simulink model "EngDem_TrqLimCoord"  (R2016b)
settings: configuration reference "CodeGenConfigSet" (kept outside this file)
values from neighbouring files (symbols this model uses):
  EngDem_facAdj_C = Calibration.Parameter    [init_EngDem_TrqLimCoord.m]    (also in init_EngDem_TrqLimCoord_SIL.m = Simulink.Parameter)
  EngDem_facAdjMax_C = Calibration.Parameter    [init_EngDem_TrqLimCoord.m]    (also in init_EngDem_TrqLimCoord_SIL.m = Simulink.Parameter)
  EngDem_facAdjMin_C = Calibration.Parameter    [init_EngDem_TrqLimCoord.m]    (also in init_EngDem_TrqLimCoord_SIL.m = Simulink.Parameter)
  EngDem_facDvolPT1_C = Calibration.Parameter    [init_EngDem_TrqLimCoord.m]    (also in init_EngDem_TrqLimCoord_SIL.m = Simulink.Parameter)
  EngDem_facResFlowPT1_C = Calibration.Parameter    [init_EngDem_TrqLimCoord.m]    (also in init_EngDem_TrqLimCoord_SIL.m = Simulink.Parameter)
  EngDem_RmpLimErrNeg_C = Calibration.Parameter    [init_EngDem_TrqLimCoord.m]    (also in init_EngDem_TrqLimCoord_SIL.m = Simulink.Parameter)
  EngDem_RmpLimErrPos_C = Calibration.Parameter    [init_EngDem_TrqLimCoord.m]    (also in init_EngDem_TrqLimCoord_SIL.m = Simulink.Parameter)
  EngDem_trqLimErr1_CUR = Calibration.Parameter    [init_EngDem_TrqLimCoord.m]    (also in init_EngDem_TrqLimCoord_SIL.m = Simulink.Parameter)
  EngDem_trqLimErr1_CURX = Calibration.Parameter    [init_EngDem_TrqLimCoord.m]    (also in init_EngDem_TrqLimCoord_SIL.m = Simulink.Parameter)
  EngDem_trqLimErr2_CUR = Calibration.Parameter    [init_EngDem_TrqLimCoord.m]    (also in init_EngDem_TrqLimCoord_SIL.m = Simulink.Parameter)
  EngDem_trqLimErr2_CURX = Calibration.Parameter    [init_EngDem_TrqLimCoord.m]    (also in init_EngDem_TrqLimCoord_SIL.m = Simulink.Parameter)
  EngDem_trqLimErr3_CUR = Calibration.Parameter    [init_EngDem_TrqLimCoord.m]    (also in init_EngDem_TrqLimCoord_SIL.m = Simulink.Parameter)
  EngDem_trqLimErr3_CURX = Calibration.Parameter    [init_EngDem_TrqLimCoord.m]    (also in init_EngDem_TrqLimCoord_SIL.m = Simulink.Parameter)
  EngDem_trqLimErr4_CUR = Calibration.Parameter    [init_EngDem_TrqLimCoord.m]    (also in init_EngDem_TrqLimCoord_SIL.m = Simulink.Parameter)
  EngDem_trqLimErr4_CURX = Calibration.Parameter    [init_EngDem_TrqLimCoord.m]    (also in init_EngDem_TrqLimCoord_SIL.m = Simulink.Parameter)
  EngDem_TrqLimErrRmpNeg_C = Calibration.Parameter    [init_EngDem_TrqLimCoord.m]    (also in init_EngDem_TrqLimCoord_SIL.m = Simulink.Parameter)
  EngDem_TrqLimErrRmpPos_C = Calibration.Parameter    [init_EngDem_TrqLimCoord.m]    (also in init_EngDem_TrqLimCoord_SIL.m = Simulink.Parameter)
  EngDem_trqLimPDiff_CUR = Calibration.Parameter    [init_EngDem_TrqLimCoord.m]    (also in init_EngDem_TrqLimCoord_SIL.m = Simulink.Parameter)
  EngDem_trqLimPDiff_CURX = Calibration.Parameter    [init_EngDem_TrqLimCoord.m]    (also in init_EngDem_TrqLimCoord_SIL.m = Simulink.Parameter)
  TRQ_MAX = fi(1000,Trq_Nm)    [init_EngDem_TrqLimCoord.m]    (also in init_EngDem_TrqLimCoord_SIL.m)
undefined symbols (not defined in the file or in its folder): CEngDsT_tTransf_CURX, EngDem_TrqLimCoord_DT
libraries: CXLib x9, simulink x1
settings Model: Creator=Administrator  LastModifiedBy=bianxuyin
settings ConfigSetRef: SourceLocation=Base Workspace

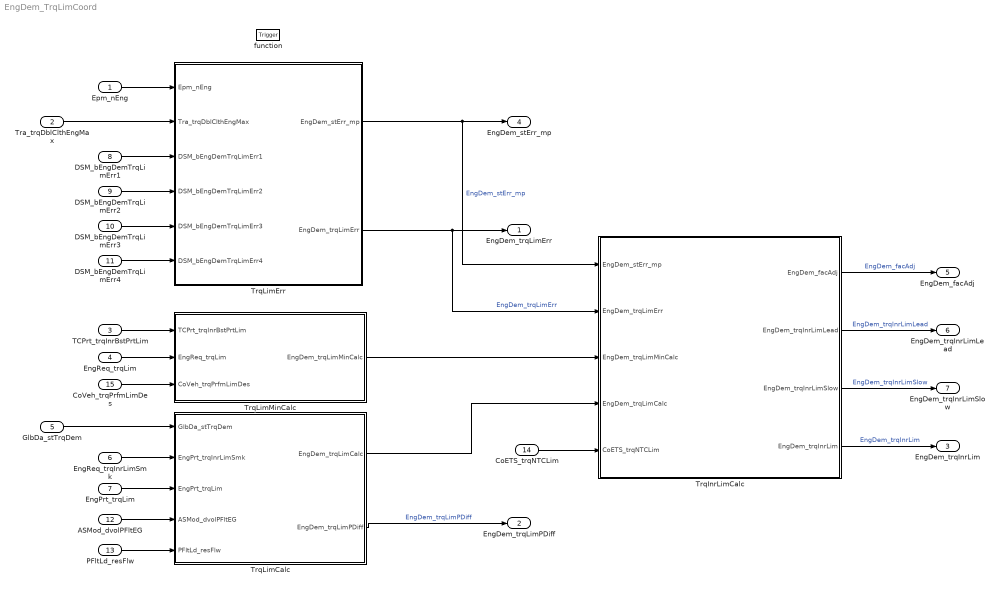
== system EngDem_TrqLimCoord ==
  Epm_nEng : Inport  Tag=rpm  Description=Engine speed  OutMin=0  OutMax=6000  OutDataTypeStr=EngSpeed_rpm
  Tra_trqDblClthEngMax : Inport  Tag=Nm  Description=Application parameter for minimum torque of systemdegratation Nm  Port=2  OutMin=-3000  OutMax=3000  OutDataTypeStr=Trq_Nm
  TCPrt_trqInrBstPrtLim : Inport  Tag=Nm  Description=Torque limitation from VGT Nm  Port=3  OutMin=-3276.8  OutMax=3276.7  OutDataTypeStr=Trq_Nm
  EngReq_trqLim : Inport  Tag=Nm  Description=Resulting limiting torque from engine specifications  Port=4  OutMin=-3276.8  OutMax=3276.7  OutDataTypeStr=Trq_Nm
  GlbDa_stTrqDem : Inport  Description=contains highest prior function with torque demand  Port=5  OutMin=0  OutMax=4294967295  OutDataTypeStr=State_uint32
  EngReq_trqInrLimSmk : Inport  Tag=Nm  Description=Limiting torque smoke limit  Port=6  OutMin=-3276.8  OutMax=3276.7  OutDataTypeStr=Trq_Nm
  EngPrt_trqLim : Inport  Tag=Nm  Description=Limitation torque for engine mechanic protection by torque limitation (as inner engine torque)  Port=7  OutMin=-3276.8  OutMax=3276.7  OutDataTypeStr=Trq_Nm
  DSM_bEngDemTrqLimErr1 : Inport  Description=FId for Engine demand Torque Limitation due to System error  Port=8  OutMin=0  OutMax=1  OutDataTypeStr=boolean
  DSM_bEngDemTrqLimErr2 : Inport  Description=FId for Engine demand Torque Limitation due to System error  Port=9  OutMin=0  OutMax=1  OutDataTypeStr=boolean
  DSM_bEngDemTrqLimErr3 : Inport  Description=FId for Engine demand Torque Limitation due to System error  Port=10  OutMin=0  OutMax=1  OutDataTypeStr=boolean
  DSM_bEngDemTrqLimErr4 : Inport  Description=FId for Engine demand Torque Limitation due to System error  Port=11  OutMin=0  OutMax=1  OutDataTypeStr=boolean
  ASMod_dvolPFltEG : Inport  Tag=m^3/h  Description=Calculated exhaust-gas volume flow in the particulate filter  Port=12  OutMin=0  OutMax=100  OutDataTypeStr=AirVol_m3_h
  PFltLd_resFlw : Inport  Tag=kPa/(m^3/h)  Description=Flow resistance of the particulate filter  Port=13  OutMin=-0.3  OutMax=0.3  OutDataTypeStr=FlowRes_kPa_m3_h
  CoETS_trqNTCLim : Inport  Tag=Nm  Description=NTC torque limitation (0 in braking, ramped to max in braked to fired  Port=14  OutMin=0  OutMax=1000  OutDataTypeStr=Trq_Nm
  CoVeh_trqPrfmLimDes : Inport  Tag=Nm  Description=Torque limitation from performence limiter  Port=15  OutMin=-3000  OutMax=3276.7  OutDataTypeStr=Trq_Nm
  function : TriggerPort  TriggerType=function-call  VariantControl=Variant
  TrqInrLimCalc : Subsystem
  TrqLimCalc : Subsystem  RTWFcnName=TrqLimCalc_Co  RTWFileName=TrqLimCalc
      settings: RTWSystemCode=Nonreusable function  RTWFcnNameOpts=User specified  RTWFileNameOpts=User specified
  TrqLimErr : Subsystem  RTWFcnName=TrqLimErr_Co  RTWFileName=TrqLimErr
      settings: RTWSystemCode=Nonreusable function  RTWFcnNameOpts=User specified  RTWFileNameOpts=User specified
  TrqLimMinCalc : Subsystem  RTWFcnName=TrqLimMinCalc_Co  RTWFileName=TrqLimMinCalc
      settings: RTWSystemCode=Nonreusable function  RTWFcnNameOpts=User specified  RTWFileNameOpts=User specified
  EngDem_trqLimErr : Outport  Tag=Nm  Description=Substitute limiting torque in the event of an error  OutMin=-3276.8  OutMax=3276.7  OutDataTypeStr=Trq_Nm
  EngDem_trqLimPDiff : Outport  Tag=Nm  Description=Limiting torque due to exhaust gas back-pressure  Port=2  OutMin=-3276.8  OutMax=3276.7  OutDataTypeStr=Trq_Nm
  EngDem_trqInrLim : Outport  Tag=Nm  Description=Resulting limiting torque (inner engine torque)  Port=3  OutMin=-3276.8  OutMax=3276.7  OutDataTypeStr=Trq_Nm
  EngDem_stErr_mp : Outport  Description=Status of the limitation FIDs  Port=4  OutMin=0  OutMax=1  OutDataTypeStr=boolean
  EngDem_facAdj : Outport  Description=EEPROM adjustment value for correction of the limiting torque  Port=5  OutMin=-10  OutMax=10  OutDataTypeStr=Factor
  EngDem_trqInrLimLead : Outport  Tag=Nm  Description=inner engine limted lead torque  Port=6  OutMin=-3276.8  OutMax=3276.7  OutDataTypeStr=Trq_Nm
  EngDem_trqInrLimSlow : Outport  Tag=Nm  Description=inner engine limted torque for Slow Path  Port=7  OutMin=-3276.8  OutMax=3276.7  OutDataTypeStr=Trq_Nm
  wires:
  TrqLimCalc/2(EngDem_trqLimPDiff) -> EngDem_trqLimPDiff/1  "EngDem_trqLimPDiff"
  Epm_nEng/1 -> TrqLimErr/1(Epm_nEng)
  Tra_trqDblClthEngMax/1 -> TrqLimErr/2(Tra_trqDblClthEngMax)
  TCPrt_trqInrBstPrtLim/1 -> TrqLimMinCalc/1(TCPrt_trqInrBstPrtLim)
  EngReq_trqLim/1 -> TrqLimMinCalc/2(EngReq_trqLim)
  GlbDa_stTrqDem/1 -> TrqLimCalc/1(GlbDa_stTrqDem)
  EngReq_trqInrLimSmk/1 -> TrqLimCalc/2(EngPrt_trqInrLimSmk)
  EngPrt_trqLim/1 -> TrqLimCalc/3(EngPrt_trqLim)
  DSM_bEngDemTrqLimErr1/1 -> TrqLimErr/3(DSM_bEngDemTrqLimErr1)
  DSM_bEngDemTrqLimErr2/1 -> TrqLimErr/4(DSM_bEngDemTrqLimErr2)
  DSM_bEngDemTrqLimErr3/1 -> TrqLimErr/5(DSM_bEngDemTrqLimErr3)
  DSM_bEngDemTrqLimErr4/1 -> TrqLimErr/6(DSM_bEngDemTrqLimErr4)
  TrqLimErr/2(EngDem_trqLimErr) -> EngDem_trqLimErr/1, TrqInrLimCalc/2(EngDem_trqLimErr)  "EngDem_trqLimErr"
  TrqLimMinCalc/1(EngDem_trqLimMinCalc) -> TrqInrLimCalc/3(EngDem_trqLimMinCalc)
  TrqLimCalc/1(EngDem_trqLimCalc) -> TrqInrLimCalc/4(EngDem_trqLimCalc)
  TrqLimErr/1(EngDem_stErr_mp) -> EngDem_stErr_mp/1, TrqInrLimCalc/1(EngDem_stErr_mp)  "EngDem_stErr_mp"
  TrqInrLimCalc/1(EngDem_facAdj) -> EngDem_facAdj/1  "EngDem_facAdj"
  TrqInrLimCalc/4(EngDem_trqInrLim) -> EngDem_trqInrLim/1  "EngDem_trqInrLim"
  TrqInrLimCalc/3(EngDem_trqInrLimSlow) -> EngDem_trqInrLimSlow/1  "EngDem_trqInrLimSlow"
  TrqInrLimCalc/2(EngDem_trqInrLimLead) -> EngDem_trqInrLimLead/1  "EngDem_trqInrLimLead"
  CoVeh_trqPrfmLimDes/1 -> TrqLimMinCalc/3(CoVeh_trqPrfmLimDes)
  ASMod_dvolPFltEG/1 -> TrqLimCalc/4(ASMod_dvolPFltEG)
  PFltLd_resFlw/1 -> TrqLimCalc/5(PFltLd_resFlw)
  CoETS_trqNTCLim/1 -> TrqInrLimCalc/5(CoETS_trqNTCLim)

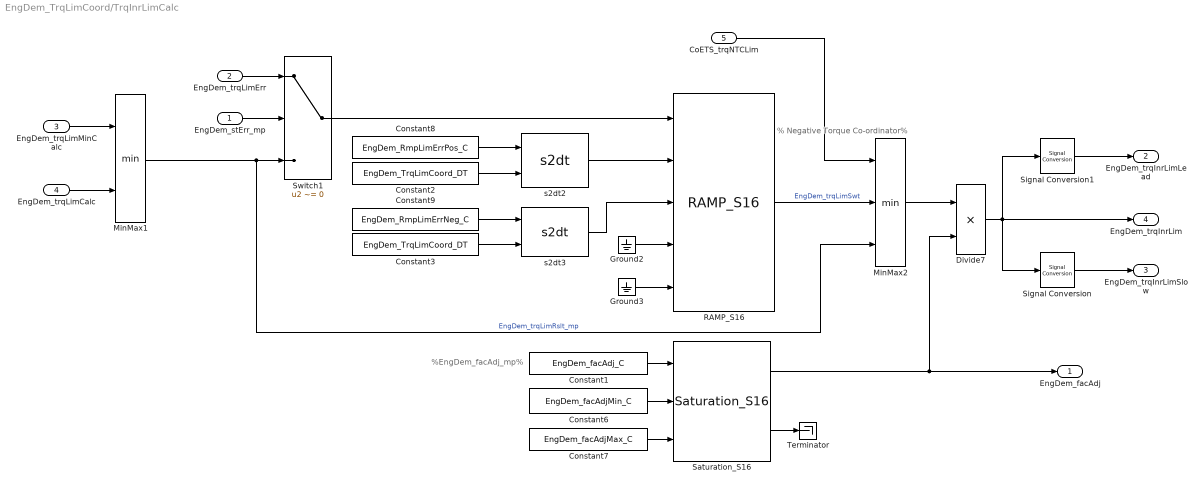
== system EngDem_TrqLimCoord/TrqInrLimCalc ==
  note: % Negative Torque Co-ordinator%
  note: %EngDem_facAdj_mp%
  EngDem_stErr_mp : Inport
  EngDem_trqLimErr : Inport  Port=2
  EngDem_trqLimMinCalc : Inport  Port=3
  EngDem_trqLimCalc : Inport  Port=4
  CoETS_trqNTCLim : Inport  Tag=Nm  Description=NTC torque limitation (0 in braking, ramped to max in braked to fired  Port=5
  Constant1 : Constant  Value=EngDem_facAdj_C
  Constant2 : Constant  Value=EngDem_TrqLimCoord_DT  OutDataTypeStr=Inherit: Inherit via back propagation
  Constant3 : Constant  Value=EngDem_TrqLimCoord_DT  OutDataTypeStr=Inherit: Inherit via back propagation
  Constant6 : Constant  Value=EngDem_facAdjMin_C
  Constant7 : Constant  Value=EngDem_facAdjMax_C
  Constant8 : Constant  Value=EngDem_RmpLimErrPos_C
  Constant9 : Constant  Value=EngDem_RmpLimErrNeg_C
  Divide7 : Product  Inputs=**  OutDataTypeStr=Trq_Nm
  Ground2 : Ground
  Ground3 : Ground
  MinMax1 : MinMax  Inputs=2  InputSameDT=on
  MinMax2 : MinMax  Inputs=3  InputSameDT=on
  RAMP_S16 : CXLib/RAMP_S16
  Saturation_S16 : CXLib/Saturation_S16
  Signal Conversion : SignalConversion  OverrideOpt=off
  Signal Conversion1 : SignalConversion  OverrideOpt=off
  Switch1 : Switch  Criteria=u2 ~= 0  InputSameDT=on
  Terminator : Terminator
  s2dt2 : CXLib/s2dt
  s2dt3 : CXLib/s2dt
  EngDem_facAdj : Outport
  EngDem_trqInrLimLead : Outport  Port=2
  EngDem_trqInrLimSlow : Outport  Port=3
  EngDem_trqInrLim : Outport  Port=4
  wires:
  Ground2/1 -> RAMP_S16/4
  MinMax2/1 -> Divide7/1
  MinMax1/1 -> MinMax2/3, Switch1/3  "EngDem_trqLimRslt_mp"
  EngDem_trqLimCalc/1 -> MinMax1/2
  Constant1/1 -> Saturation_S16/1
  Ground3/1 -> RAMP_S16/5
  Constant6/1 -> Saturation_S16/2
  CoETS_trqNTCLim/1 -> MinMax2/1
  EngDem_trqLimMinCalc/1 -> MinMax1/1
  Saturation_S16/2 -> Terminator/1
  Constant7/1 -> Saturation_S16/3
  Saturation_S16/1 -> EngDem_facAdj/1, Divide7/2
  RAMP_S16/1 -> MinMax2/2  "EngDem_trqLimSwt"
  Constant9/1 -> s2dt3/1
  Constant8/1 -> s2dt2/1
  Switch1/1 -> RAMP_S16/1
  EngDem_trqLimErr/1 -> Switch1/1
  EngDem_stErr_mp/1 -> Switch1/2
  s2dt2/1 -> RAMP_S16/2
  Constant2/1 -> s2dt2/2
  s2dt3/1 -> RAMP_S16/3
  Constant3/1 -> s2dt3/2
  Divide7/1 -> EngDem_trqInrLim/1, Signal Conversion/1, Signal Conversion1/1
  Signal Conversion1/1 -> EngDem_trqInrLimLead/1
  Signal Conversion/1 -> EngDem_trqInrLimSlow/1

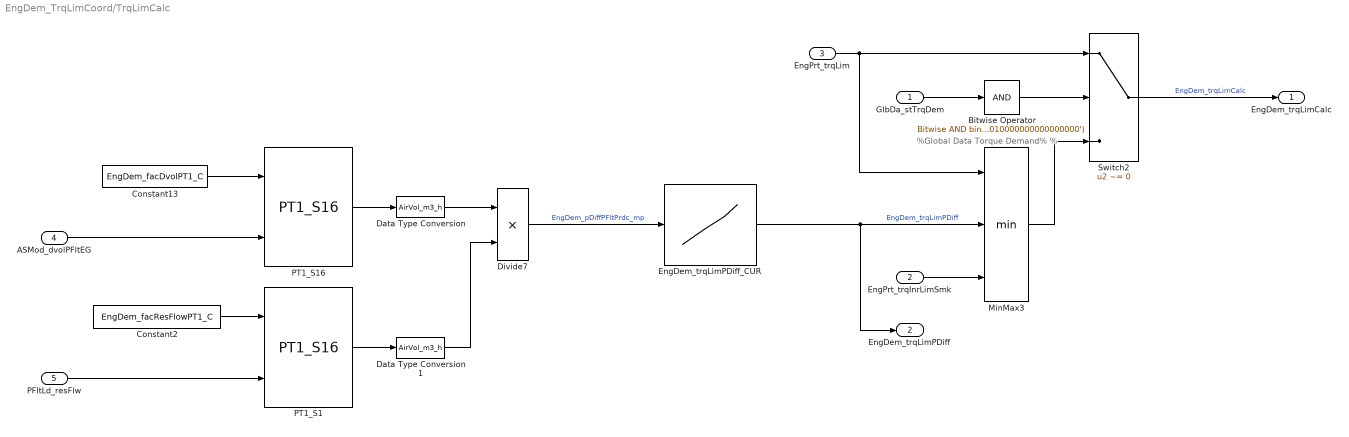
== system EngDem_TrqLimCoord/TrqLimCalc ==
  note: %Global Data Torque Demand% %
  GlbDa_stTrqDem : Inport
  EngPrt_trqInrLimSmk : Inport  Port=2
  EngPrt_trqLim : Inport  Port=3
  ASMod_dvolPFltEG : Inport  Tag=m^2/h  Description=Calculated exhaust-gas volume flow in the particulate filter  Port=4
  PFltLd_resFlw : Inport  Tag=kPa/(m^2/h)  Description=Flow resistance of the particulate filter  Port=5
  " EngDem_trqLimPDiff_CUR" : Lookup_n-D  DialogController=Simulink.DDGSource  NumberOfTableDimensions=1  BreakpointsForDimension1=EngDem_trqLimPDiff_CURX  BreakpointsForDimension2=CEngDsT_tTransf_CURX  IndexSearchMethod=Linear search  BeginIndexSearchUsingPreviousIndexResult=on  Table=EngDem_trqLimPDiff_CUR  ExtrapMethod=Clip  UseLastTableValue=on  InternalRulePriority=Speed  OutDataTypeStr=Inherit: Inherit via back propagation  SaturateOnIntegerOverflow=on
  Bitwise Operator : simulink/Logic and Bit Operations/Bitwise Operator  logicop=AND  UseBitMask=on  BitMask=bin2dec('00000000000000010000000000000000')  BitMaskRealWorld=Stored Integer
  Constant13 : Constant  Value=EngDem_facDvolPT1_C
  Constant2 : Constant  Value=EngDem_facResFlowPT1_C
  Data Type Conversion : DataTypeConversion  OutDataTypeStr=AirVol_m3_h  RndMeth=Round  SaturateOnIntegerOverflow=on
  Data Type Conversion1 : DataTypeConversion  OutDataTypeStr=AirVol_m3_h  RndMeth=Round  SaturateOnIntegerOverflow=on
  Divide7 : Product  Inputs=**  OutDataTypeStr=AirPressure_kPa
  MinMax3 : MinMax  Inputs=3  InputSameDT=on
  PT1_S1 : CXLib/PT1_S16
  PT1_S16 : CXLib/PT1_S16
  Switch2 : Switch  Criteria=u2 ~= 0  InputSameDT=on
  EngDem_trqLimCalc : Outport
  EngDem_trqLimPDiff : Outport  Port=2
  wires:
  GlbDa_stTrqDem/1 -> Bitwise Operator/1
  EngPrt_trqLim/1 -> MinMax3/1, Switch2/1
  MinMax3/1 -> Switch2/3
  " EngDem_trqLimPDiff_CUR"/1 -> EngDem_trqLimPDiff/1, MinMax3/2  "EngDem_trqLimPDiff"
  Divide7/1 -> " EngDem_trqLimPDiff_CUR"/1  "EngDem_pDiffPFltPrdc_mp"
  ASMod_dvolPFltEG/1 -> PT1_S16/2
  EngPrt_trqInrLimSmk/1 -> MinMax3/3
  Switch2/1 -> EngDem_trqLimCalc/1  "EngDem_trqLimCalc"
  Constant13/1 -> PT1_S16/1
  Constant2/1 -> PT1_S1/1
  Bitwise Operator/1 -> Switch2/2
  PT1_S16/1 -> Data Type Conversion/1
  PFltLd_resFlw/1 -> PT1_S1/2
  PT1_S1/1 -> Data Type Conversion1/1
  Data Type Conversion1/1 -> Divide7/2
  Data Type Conversion/1 -> Divide7/1

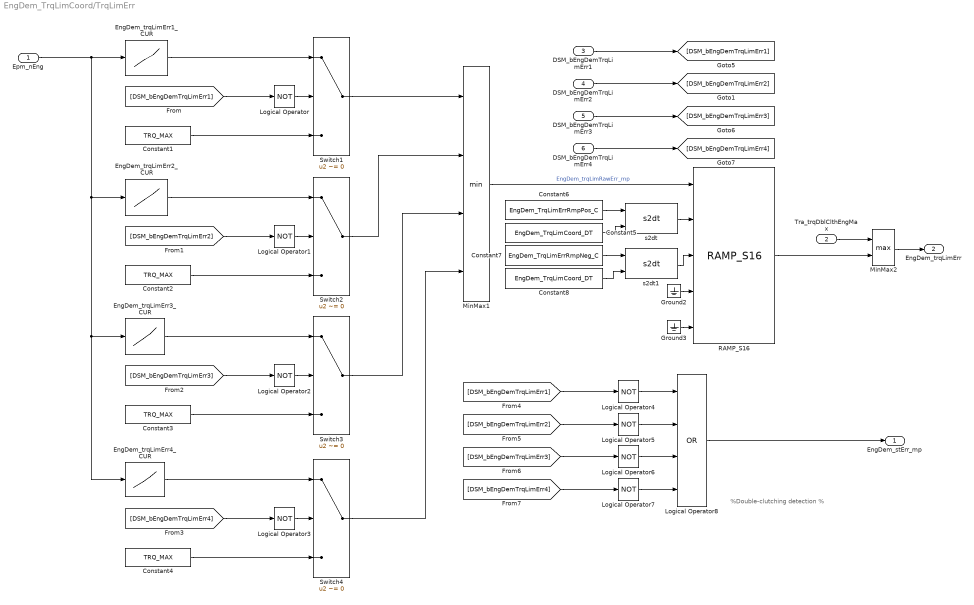
== system EngDem_TrqLimCoord/TrqLimErr ==
  note: %Double-clutching detection %
  Epm_nEng : Inport  Description=Engine speed
  Tra_trqDblClthEngMax : Inport  Port=2
  DSM_bEngDemTrqLimErr1 : Inport  Description=status of FId_EngDemTrqLimErr1  Port=3  OutMin=0  OutMax=1  OutDataTypeStr=boolean
  DSM_bEngDemTrqLimErr2 : Inport  Description=status of FId_EngDemTrqLimErr2  Port=4  OutMin=0  OutMax=1  OutDataTypeStr=boolean
  DSM_bEngDemTrqLimErr3 : Inport  Description=status of FId_EngDemTrqLimErr3  Port=5  OutMin=0  OutMax=1  OutDataTypeStr=boolean
  DSM_bEngDemTrqLimErr4 : Inport  Description=status of FId_EngDemTrqLimErr4  Port=6  OutMin=0  OutMax=1  OutDataTypeStr=boolean
  " EngDem_trqLimErr1_CUR" : Lookup_n-D  DialogController=Simulink.DDGSource  NumberOfTableDimensions=1  BreakpointsForDimension1=EngDem_trqLimErr1_CURX  BreakpointsForDimension2=CEngDsT_tTransf_CURX  IndexSearchMethod=Linear search  BeginIndexSearchUsingPreviousIndexResult=on  Table=EngDem_trqLimErr1_CUR  ExtrapMethod=Clip  UseLastTableValue=on  InternalRulePriority=Speed  OutDataTypeStr=Inherit: Inherit via back propagation  SaturateOnIntegerOverflow=on
  " EngDem_trqLimErr2_CUR" : Lookup_n-D  DialogController=Simulink.DDGSource  NumberOfTableDimensions=1  BreakpointsForDimension1=EngDem_trqLimErr2_CURX  BreakpointsForDimension2=CEngDsT_tTransf_CURX  IndexSearchMethod=Linear search  BeginIndexSearchUsingPreviousIndexResult=on  Table=EngDem_trqLimErr2_CUR  ExtrapMethod=Clip  UseLastTableValue=on  InternalRulePriority=Speed  OutDataTypeStr=Inherit: Inherit via back propagation  SaturateOnIntegerOverflow=on
  " EngDem_trqLimErr3_CUR" : Lookup_n-D  DialogController=Simulink.DDGSource  NumberOfTableDimensions=1  BreakpointsForDimension1=EngDem_trqLimErr3_CURX  BreakpointsForDimension2=CEngDsT_tTransf_CURX  IndexSearchMethod=Linear search  BeginIndexSearchUsingPreviousIndexResult=on  Table=EngDem_trqLimErr3_CUR  ExtrapMethod=Clip  UseLastTableValue=on  InternalRulePriority=Speed  OutDataTypeStr=Inherit: Inherit via back propagation  SaturateOnIntegerOverflow=on
  " EngDem_trqLimErr4_CUR" : Lookup_n-D  DialogController=Simulink.DDGSource  NumberOfTableDimensions=1  BreakpointsForDimension1=EngDem_trqLimErr4_CURX  BreakpointsForDimension2=CEngDsT_tTransf_CURX  IndexSearchMethod=Linear search  BeginIndexSearchUsingPreviousIndexResult=on  Table=EngDem_trqLimErr4_CUR  ExtrapMethod=Clip  UseLastTableValue=on  InternalRulePriority=Speed  OutDataTypeStr=Inherit: Inherit via back propagation  SaturateOnIntegerOverflow=on
  Constant{1..4} (4 alike) : Constant  Value=TRQ_MAX  OutDataTypeStr=Trq_Nm
  Constant5 : Constant  Value=EngDem_TrqLimCoord_DT  OutDataTypeStr=Inherit: Inherit via back propagation
  Constant6 : Constant  Value=EngDem_TrqLimErrRmpPos_C
  Constant7 : Constant  Value=EngDem_TrqLimErrRmpNeg_C
  Constant8 : Constant  Value=EngDem_TrqLimCoord_DT  OutDataTypeStr=Inherit: Inherit via back propagation
  Ground2 : Ground
  Ground3 : Ground
  Logical Operator{,1..7} (8 alike) : Logic  Operator=NOT  AllPortsSameDT=off  OutDataTypeStr=boolean
  Logical Operator8 : Logic  Operator=OR  Inputs=4  AllPortsSameDT=off  OutDataTypeStr=boolean
  MinMax1 : MinMax  Inputs=4  InputSameDT=on
  MinMax2 : MinMax  Function=max  Inputs=2  InputSameDT=on
  RAMP_S16 : CXLib/RAMP_S16
  Switch{1..4} (4 alike) : Switch  Criteria=u2 ~= 0  InputSameDT=on
  s2dt : CXLib/s2dt
  s2dt1 : CXLib/s2dt
  EngDem_stErr_mp : Outport
  EngDem_trqLimErr : Outport  Port=2
  wires:
  MinMax1/1 -> RAMP_S16/1  "EngDem_trqLimRawErr_mp"
  Switch1/1 -> MinMax1/1
  Logical Operator/1 -> Switch1/2
  [DSM_bEngDemTrqLimErr1] -> Logical Operator/1
  " EngDem_trqLimErr1_CUR"/1 -> Switch1/1
  Logical Operator1/1 -> Switch2/2
  [DSM_bEngDemTrqLimErr2] -> Logical Operator1/1
  " EngDem_trqLimErr2_CUR"/1 -> Switch2/1
  Switch2/1 -> MinMax1/2
  Logical Operator2/1 -> Switch3/2
  [DSM_bEngDemTrqLimErr3] -> Logical Operator2/1
  " EngDem_trqLimErr3_CUR"/1 -> Switch3/1
  Switch3/1 -> MinMax1/3
  Logical Operator3/1 -> Switch4/2
  [DSM_bEngDemTrqLimErr4] -> Logical Operator3/1
  " EngDem_trqLimErr4_CUR"/1 -> Switch4/1
  Switch4/1 -> MinMax1/4
  Epm_nEng/1 -> " EngDem_trqLimErr4_CUR"/1, " EngDem_trqLimErr3_CUR"/1, " EngDem_trqLimErr2_CUR"/1, " EngDem_trqLimErr1_CUR"/1
  Ground2/1 -> RAMP_S16/4
  Ground3/1 -> RAMP_S16/5
  Tra_trqDblClthEngMax/1 -> MinMax2/1
  Logical Operator4/1 -> Logical Operator8/1
  Logical Operator5/1 -> Logical Operator8/2
  Logical Operator6/1 -> Logical Operator8/3
  Logical Operator7/1 -> Logical Operator8/4
  Constant6/1 -> s2dt/1
  Constant7/1 -> s2dt1/1
  RAMP_S16/1 -> MinMax2/2
  Logical Operator8/1 -> EngDem_stErr_mp/1
  Constant1/1 -> Switch1/3
  Constant2/1 -> Switch2/3
  Constant3/1 -> Switch3/3
  Constant4/1 -> Switch4/3
  DSM_bEngDemTrqLimErr1/1 -> [DSM_bEngDemTrqLimErr1]
  DSM_bEngDemTrqLimErr2/1 -> [DSM_bEngDemTrqLimErr2]
  DSM_bEngDemTrqLimErr3/1 -> [DSM_bEngDemTrqLimErr3]
  DSM_bEngDemTrqLimErr4/1 -> [DSM_bEngDemTrqLimErr4]
  [DSM_bEngDemTrqLimErr1] -> Logical Operator4/1
  [DSM_bEngDemTrqLimErr2] -> Logical Operator5/1
  [DSM_bEngDemTrqLimErr3] -> Logical Operator6/1
  [DSM_bEngDemTrqLimErr4] -> Logical Operator7/1
  MinMax2/1 -> EngDem_trqLimErr/1
  s2dt/1 -> RAMP_S16/2
  s2dt1/1 -> RAMP_S16/3
  Constant5/1 -> s2dt/2
  Constant8/1 -> s2dt1/2

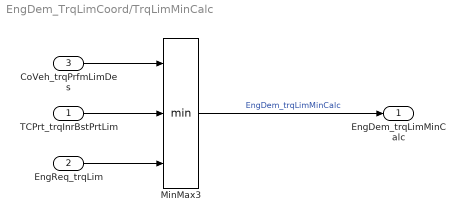
== system EngDem_TrqLimCoord/TrqLimMinCalc ==
  TCPrt_trqInrBstPrtLim : Inport
  EngReq_trqLim : Inport  Port=2
  CoVeh_trqPrfmLimDes : Inport  Tag=Nm  Description=Torque limitation from performence limiter  Port=3
  MinMax3 : MinMax  Inputs=3  InputSameDT=on
  EngDem_trqLimMinCalc : Outport
  wires:
  CoVeh_trqPrfmLimDes/1 -> MinMax3/1
  TCPrt_trqInrBstPrtLim/1 -> MinMax3/2
  EngReq_trqLim/1 -> MinMax3/3
  MinMax3/1 -> EngDem_trqLimMinCalc/1  "EngDem_trqLimMinCalc"
